simulink model "test"  (R2013a)
settings: Solver=ode45  StartTime=0.0  StopTime=1  RelTol=1e-3
settings Model: Creator=sebastian  LastModifiedBy=sebastian

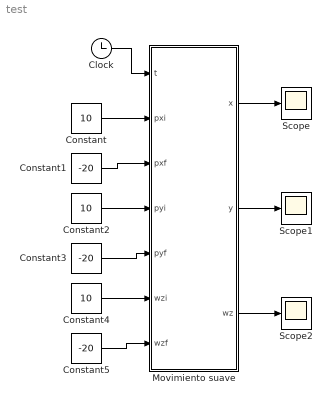
== system test ==
  Clock : Clock
  Constant : Constant  Value=10
  Constant1 : Constant  Value=-20
  Constant2 : Constant  Value=10
  Constant3 : Constant  Value=-20
  Constant4 : Constant  Value=10
  Constant5 : Constant  Value=-20
  Movimiento suave : MATLAB Function  TreatAsAtomicUnit=on
  Scope : Scope
  Scope1 : Scope
  Scope2 : Scope
      settings: SaveName=ScopeData2
  wires:
  Clock/1 -> Movimiento suave/1(t)
  Movimiento suave/1(x) -> Scope/1
  Constant/1 -> Movimiento suave/2(pxi)
  Constant1/1 -> Movimiento suave/3(pxf)
  Movimiento suave/2(y) -> Scope1/1
  Movimiento suave/3(wz) -> Scope2/1
  Constant2/1 -> Movimiento suave/4(pyi)
  Constant3/1 -> Movimiento suave/5(pyf)
  Constant4/1 -> Movimiento suave/6(wzi)
  Constant5/1 -> Movimiento suave/7(wzf)

== matlab function test/Movimiento suave ==
  data: t input; x output; pxi input; pxf input; pyi input; pyf input; wzi input; wzf input; y output; wz output
function [x,y,wz]= fcn(t,pxi,pxf,pyi,pyf,wzi,wzf)

x = pxi + 3*(pxf-pxi)*t^2 - 2*(pxf-pxi)*t^3;
y = pyi + 3*(pyf-pyi)*t^2 - 2*(pyf-pyi)*t^3;
wz = wzi + 3*(wzf-wzi)*t^2 - 2*(wzf-wzi)*t^3;
